simulink model "L3_Q2_Sim"  (R2015a)
settings: Solver=ode3  StartTime=0.0  StopTime=tf  FixedStep=t_step  RelTol=1e-3
values from neighbouring files (symbols this model uses):
  a = 0.01    [L3_Q1.m]    (also in L3_Q2.m)
  a0_hat = 0.02    [L3_Q1.m]    (also in L3_Q2.m)
  alpha = 10    [L3_Q2.m]
  b = 2    [L3_Q1.m]    (also in L3_Q2.m)
  b0_hat = 1    [L3_Q1.m]    (also in L3_Q2.m)
  K0 = -log(0.01)/0.5    [L3_Q1.m]    (also in L3_Q2.m)
  lf = 3    [L3_Q2.m]
  T_ref = 2    [L3_Q1.m]    (also in L3_Q2.m)
settings Model: Creator=Marcelo  LastModifiedBy=Marcelo

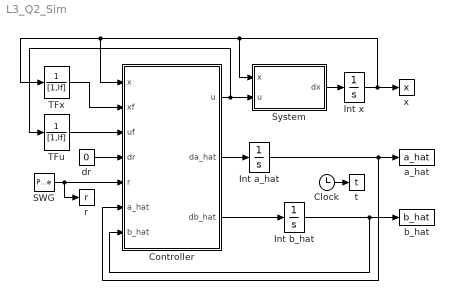
== system L3_Q2_Sim ==
  Clock : Clock
  Controller : MATLAB Function  TreatAsAtomicUnit=on
  Int a_hat : Integrator  InitialCondition=a0_hat
  Int b_hat : Integrator  InitialCondition=b0_hat
  Int x : Integrator
  SWG : DiscretePulseGenerator  PulseType=Time based  Period=T_ref  PulseWidth=50
  System : MATLAB Function  TreatAsAtomicUnit=on
  TFu : TransferFcn  Denominator=[1,lf]
  TFx : TransferFcn  Denominator=[1,lf]
  a_hat : ToWorkspace  VariableName=a_hat  SampleTime=-1
  b_hat : ToWorkspace  VariableName=b_hat  SampleTime=-1
  dr : Constant  Value=0
  r : ToWorkspace  VariableName=r  SampleTime=-1
  t : ToWorkspace  VariableName=t  SampleTime=-1
  x : ToWorkspace  VariableName=x  SampleTime=-1
  wires:
  System/1(dx) -> Int x/1
  Int x/1 -> x/1, System/1(x), TFx/1, Controller/1(x)
  Controller/3(db_hat) -> Int b_hat/1
  Int b_hat/1 -> b_hat/1, Controller/7(b_hat)
  Int a_hat/1 -> a_hat/1, Controller/6(a_hat)
  Clock/1 -> t/1
  SWG/1 -> Controller/5(r), r/1
  dr/1 -> Controller/4(dr)
  Controller/2(da_hat) -> Int a_hat/1
  TFu/1 -> Controller/3(uf)
  TFx/1 -> Controller/2(xf)
  Controller/1(u) -> System/2(u), TFu/1

== matlab function L3_Q2_Sim/Controller ==
  data: u output; da_hat output; x input; xf input; uf input; dr input; r input; a_hat input; b_hat input; db_hat output; alpha parameter; K0 parameter; lf parameter
function [u, da_hat, db_hat] = fcn(x, xf, uf, dr, r, a_hat, b_hat, alpha, K0, lf)
v = dr - K0 * (x - r);
u = (a_hat * x + v) / b_hat;

x_tilde = xf * (lf - a_hat) + uf * b_hat - x;
da_hat = + alpha * x_tilde * xf;
db_hat = - alpha * x_tilde * uf;

== matlab function L3_Q2_Sim/System ==
  data: x input; u input; dx output; a parameter; b parameter
function dx = fcn(x, u, a, b)
dx = -a*x + b*u;
